simulink model "TransmissionDownshift"  (R2022a)
settings: Solver=ode5  StartTime=0.0  StopTime=100  RelTol=1e-3  AbsTol=1e-6
model workspace (MAT data in the model file):
  Iei = 0.0219914882836
  converter_data = [0  137.465208994  2.232; 0.1  137.065019157  2.075; 0.2  135.864449646  1.975; 0.3  135.664354728  1.846; 0.4  137.565256453  1.72; 0.5  140.366585312  1.564; 0.6  145.268910814  1.409; 0.7  152.872517717  1.254; 0.8  162.9773111  1.096; 0.81  164.27792807  1.08; 0.82  166.178829795  1.061; 0.83  167.979684062  1.043; 0.84  170.080680706  1.028; 0.85  172.781962105  1.012; 0.86  175.383196045  1.002; 0.87  179.585189333  1.002; 0.88  183.587087703  1.001; 0.89  189.890077635  0.998; 0.9  197.693779455  0.999; 0.92  215.902417037  1.001; 0.94  244.515990379  1.002]
  downtab = [0  5  20  35; 0  5  20  35; 0  5  25  40; 0  5  30  50; 0  30  50  80; 0  30  50  80]
  downth = [0; 5; 40; 50; 90; 100]
  emap = [-40  -44  -49  -53  -57  -61  -65  -70  -74  -78  -82; 215  117  85  66  44  29  10  -2  -13  -22  -32; 245  208  178  148  122  104  85  66  48  33  18; 264  260  241  219  193  167  152  133  119  96  85; 264  279  282  275  260  238  223  208  189  171  152; 267  290  293  297  290  275  260  256  234  212  193; 267  297  305  305  305  301  293  282  267  249  226; 267  301  308  312  319  323  319  316  297  279  253; 267  301  312  319  327  327  327  327  312  293  267; 267  301  312  319  327  334  334  334  319  305  275]
  nevec = [800 1200 1600 2000 2400 2800 3200 3600 4000 4400 4800]
  p0 = 0.07934
  p1 = 0.07934
  thvec = [0; 20; 30; 40; 50; 60; 70; 80; 90; 100]
  uptab = [10  30  50  1000000; 10  30  50  1000000; 15  30  50  1000000; 23  41  60  1000000; 40  70  100  1000000; 40  70  100  1000000]
  upth = [0; 25; 35; 50; 90; 100]
  vehicledata = [3.23; 40; 0.3; 1; 50; 0]
undefined symbols (not defined in the file or in its folder): gearType, Hecate_Param1, Hecate_Param2, Hecate_Param3, Hecate_Param4
Description:
  | TransmissionDownshiftTestSequence model
  | The model is used to show how to test a transmission shift logic controller using test sequences and assessments.
settings Model: ExtModeTrigMode=oneshot  ExtModeArmWhenConnect=off  Creator=The MathWorks, Inc.  LastModifiedBy=admin
settings SolverCC: AutoScaleAbsTol=off  AlgebraicLoopSolver=TrustRegion  MaxZcPerStep=1
settings DataIOCC: InitialState=X0  LoadInitialState=on  SaveFormat=Structure  ReturnWorkspaceOutputs=off  SignalLoggingName=sigsOut
settings OptimizationCC: BlockReduction=off  BooleanDataType=off  DefaultParameterBehavior=Inlined  ExpressionDepthLimit=2147483647  InitFltsAndDblsToZero=on  EfficientMapNaN2IntZero=off  LifeSpan=1  EfficientTunableParamExpr=on
settings DebuggingCC: SaveWithParameterizedLinksMsg=none  UnderspecifiedInitializationDetection=Classic  MergeDetectMultiDrivingBlocksExec=none  CheckExecutionContextPreStartOutputMsg=on  SignalResolutionControl=TryResolveAllWithWarning  MultiTaskDSMMsg=warning  MultiTaskCondExecSysMsg=none  IntegerOverflowMsg=none  FcnCallInpInsideContextMsg=warning  UnconnectedInputMsg=warning  UnconnectedOutputMsg=warning  UnconnectedLineMsg=warning  AllowSymbolicDim=off  StateNameClashWarn=warning  SFUnexpectedBacktrackingDiag=warning  SFNoUnconditionalDefaultTransitionDiag=warning  SFExecutionAtInitializationDiag=none  SFMachineParentedDataDiag=warning  IntegerSaturationMsg=none  ArithmeticOperatorsInVariantConditions=warning
settings HardwareCC: ProdBitPerPointer=32  ProdBitPerSizeT=32  ProdBitPerPtrDiffT=32  ProdLargestAtomicFloat=None  ProdIntDivRoundTo=Undefined  ProdEndianess=Unspecified  ProdWordSize=32  ProdHWDeviceType=32-bit Generic  TargetBitPerLong=64  TargetBitPerPointer=64  TargetBitPerSizeT=64  TargetBitPerPtrDiffT=64  TargetLongLongMode=on  TargetIntDivRoundTo=Zero  TargetEndianess=LittleEndian  TargetWordSize=64  TargetHWDeviceType=MATLAB Host  ProdEqTarget=off
settings ModelReferenceCC: PropagateSignalLabelsOutOfModel=off
settings SFSimCC: SFSimEcho=off  SimUseLocalCustomCode=off  SimParseCustomCode=off  MATLABDynamicMemAlloc=off  CustomCodeUndefinedFunction=UseInterfaceOnly
settings RTWCC: SystemTargetFile=ert.tlc  TemplateMakefile=ert_default_tmf  RTWUseLocalCustomCode=off  DLArmComputeVersion=19.05
settings CodeAppCC: IgnoreCustomStorageClasses=off  CustomSymbolStrModelFcn=$N  StateflowObjectComments=on
settings ERTTargetCC: MultiwordLength=2048  GenerateSampleERTMain=on  InlinedParameterPlacement=NonHierarchical  ERTCustomFileTemplate=example_file_process.tlc  ConvertIfToSwitch=off  SuppressUnreachableDefaultCases=off
settings ConfigComp: CovMetricSettings=dcmtr  CovSaveCumulativeToWorkspaceVar=on  CovSaveSingleToWorkspaceVar=on  CovExternalEMLEnable=off  CovSFcnEnable=off

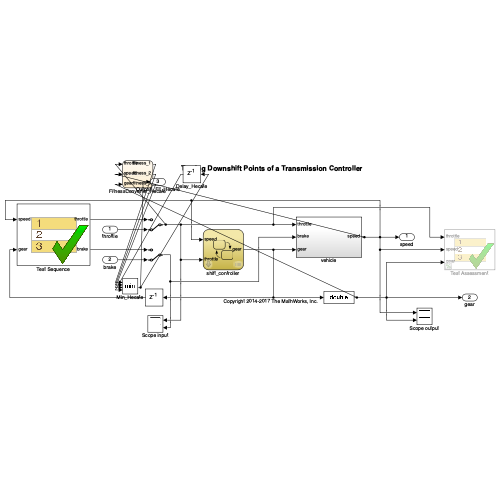
[thumbnail: Simulink's stored preview of the top-level diagram]
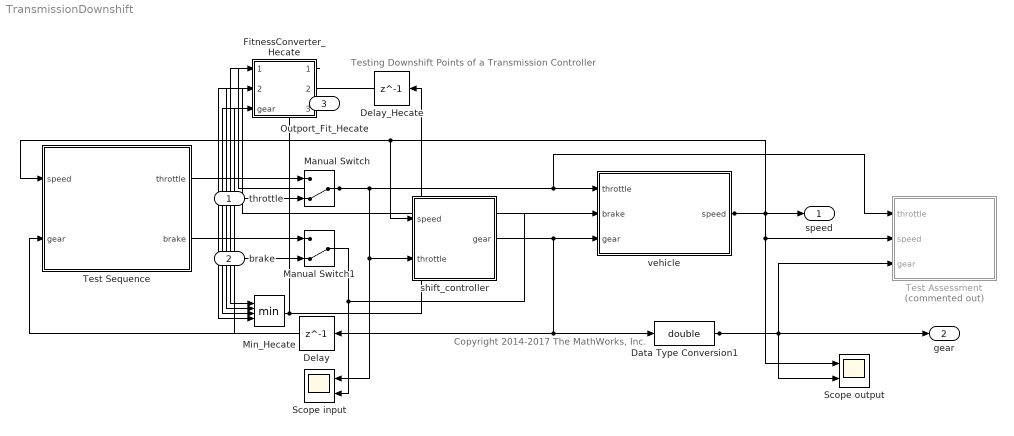
== system TransmissionDownshift ==
  note: Copyright 2014-2017 The MathWorks, Inc.
  note: Testing Downshift Points of a Transmission Controller
  throttle : Inport
  brake : Inport  Port=2
  Data Type Conversion1 : DataTypeConversion  OutDataTypeStr=double  SaturateOnIntegerOverflow=off  RndMeth=Floor
  Delay : Delay  DelayLength=1  InitialCondition=gearType.first
  Delay_Hecate : Delay  DelayLength=1  InitialCondition=Inf
  FitnessConverter_Hecate : Stateflow chart  TreatAsAtomicUnit=on
  Manual Switch : ManualSwitch  CurrentSetting=0
  Manual Switch1 : ManualSwitch  CurrentSetting=0
  Min_Hecate : MinMax  Inputs=4
  Scope input : Scope  NumInputPorts=2
  Scope output : Scope  NumInputPorts=2
  Test Assessment : Test Sequence  Tag=__SLT_ASMT__  Commented=on  TreatAsAtomicUnit=on
  Test Sequence : Test Sequence  TreatAsAtomicUnit=on
  shift_controller : Stateflow chart  TreatAsAtomicUnit=on  mask{TWAIT=2}
      mask prompts: TWAIT "Delay before gear change (tick)"
  vehicle : Subsystem
  speed : Outport  VectorParamsAs1DForOutWhenUnconnected=off
  gear : Outport  Port=2  VectorParamsAs1DForOutWhenUnconnected=off
  Outport_Fit_Hecate : Outport  Port=3
  wires:
  vehicle/1(speed) -> speed/1, Test Assessment/2(speed), Scope output/1, Test Sequence/1(speed), shift_controller/1(speed), FitnessConverter_Hecate/2(speed)
  Test Sequence/2(brake) -> Manual Switch1/1
  Test Sequence/1(throttle) -> Manual Switch/1
  throttle/1 -> Manual Switch/2
  brake/1 -> Manual Switch1/2
  Manual Switch/1 -> vehicle/1(throttle), Test Assessment/1(throttle), Scope input/1, shift_controller/2(throttle), FitnessConverter_Hecate/1(throttle)
  Manual Switch1/1 -> vehicle/2(brake), Scope input/2
  Delay/1 -> Test Sequence/2(gear)
  shift_controller/1(" gear") -> Delay/1, Data Type Conversion1/1, vehicle/3(gear)
  Data Type Conversion1/1 -> Test Assessment/3(gear), gear/1, Scope output/2, FitnessConverter_Hecate/3(gear)
  FitnessConverter_Hecate/1(fitness_1) -> Min_Hecate/1
  FitnessConverter_Hecate/2(fitness_2) -> Min_Hecate/2
  FitnessConverter_Hecate/3(fitness_3) -> Min_Hecate/3
  Min_Hecate/1 -> Delay_Hecate/1, Outport_Fit_Hecate/1
  Delay_Hecate/1 -> Min_Hecate/4

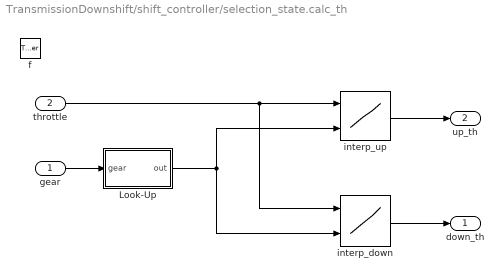
== system TransmissionDownshift/shift_controller/selection_state.calc_th ==
  gear : Inport  OutDataTypeStr=Enum: gearType  PortDimensions=1
  throttle : Inport  Port=2  OutDataTypeStr=double  PortDimensions=1
  f : TriggerPort  TriggerType=function-call  VariantControl=Variant
      settings: CopyFcn=Stateflow.SLINSF.SimulinkMan.removeBlockPreDeleteFcn  PreDeleteFcn=Stateflow.SLINSF.SimulinkMan.unsafePredeleteFcn
  Look-Up : MATLAB Function  TreatAsAtomicUnit=on
  interp_down : Lookup_n-D  BreakpointsForDimension1=downth  BreakpointsForDimension2=[1:4]  Table=downtab
      settings: InputPortMap=u0,u1
  interp_up : Lookup_n-D  BreakpointsForDimension1=upth  BreakpointsForDimension2=[1:4]  Table=uptab
      settings: InputPortMap=u0,u1
  down_th : Outport  VectorParamsAs1DForOutWhenUnconnected=off
  up_th : Outport  Port=2  VectorParamsAs1DForOutWhenUnconnected=off
  wires:
  interp_up/1 -> up_th/1
  interp_down/1 -> down_th/1
  throttle/1 -> interp_down/1, interp_up/1
  gear/1 -> Look-Up/1(gear)
  Look-Up/1(out) -> interp_down/2, interp_up/2

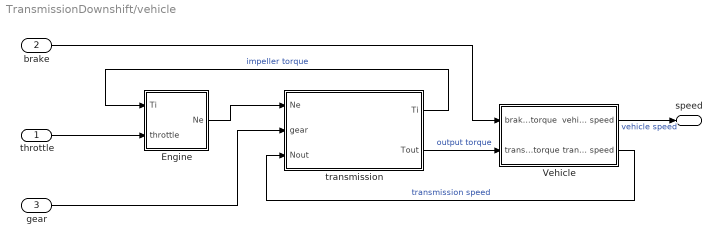
== system TransmissionDownshift/vehicle ==
  throttle : Inport
  brake : Inport  Port=2
  gear : Inport  Port=3
  Engine : Subsystem
  Vehicle : Subsystem  mask(vehicle model){Rfd=vehicledata(1), rload0=vehicledata(2), rload2=vehicledata(3), Rw=vehicledata(4), Iv=vehicledata(5), N20=vehicledata(6)/vehicledata(4)*vehicledata(1)}
      mask prompts: Rfd "final drive ratio"; rload0 "drag friction at wheels"; rload2 "aerodynamic drag"; Rw "wheel radius"; Iv "vehicle inertia"; N20 "initial transmission output speed"
      mask help: vehicle dynamics: torque input from trans., outputs are input speed (transmission output) and vehicle speed
      mask Display: image('NSX_3Colors.jpg')
  transmission : Subsystem
      mask Display:
      | image('transmission_diagram.svg')
      | port_label('input', 1, 'Ne')
      | port_label('input', 2, 'gear')
      | port_label('input', 3, 'Nout')
      | port_label('output', 1, 'Ti')
      | port_label('output', 2, 'Tout')
  speed : Outport  VectorParamsAs1DForOutWhenUnconnected=off
  wires:
  throttle/1 -> Engine/2(throttle)
  transmission/1(Ti) -> Engine/1(Ti)  "impeller torque"
  Engine/1(Ne) -> transmission/1(Ne)
  transmission/2(Tout) -> Vehicle/2(transmission output torque)  "output torque"
  Vehicle/2(transmission output speed) -> transmission/3(Nout)  "transmission speed"
  Vehicle/1(vehicle speed) -> speed/1  "vehicle speed"
  brake/1 -> Vehicle/1(brake torque)
  gear/1 -> transmission/2(gear)

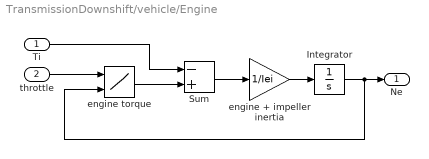
== system TransmissionDownshift/vehicle/Engine ==
  Ti : Inport
  throttle : Inport  Port=2
  Integrator : Integrator  InitialCondition=1000  LimitOutput=on  UpperSaturationLimit=6000  LowerSaturationLimit=600  ZeroCross=off
  Sum : Sum  Inputs=-+  InputSameDT=on  SaturateOnIntegerOverflow=on  OutDataTypeStr=Inherit: Same as first input
  engine torque : Lookup_n-D  BreakpointsForDimension1=thvec  BreakpointsForDimension2=nevec  Table=emap  InternalRulePriority=Speed
      settings: InputPortMap=u0,u1
  engine + impeller inertia : Gain  Gain=1/Iei  SaturateOnIntegerOverflow=on  OutDataTypeStr=Inherit: Same as input  ParamDataTypeStr=Inherit: Same as input
  Ne : Outport  VectorParamsAs1DForOutWhenUnconnected=off
  wires:
  Ti/1 -> Sum/1
  throttle/1 -> engine torque/1
  Integrator/1 -> engine torque/2, Ne/1
  Sum/1 -> engine + impeller inertia/1
  engine + impeller inertia/1 -> Integrator/1
  engine torque/1 -> Sum/2

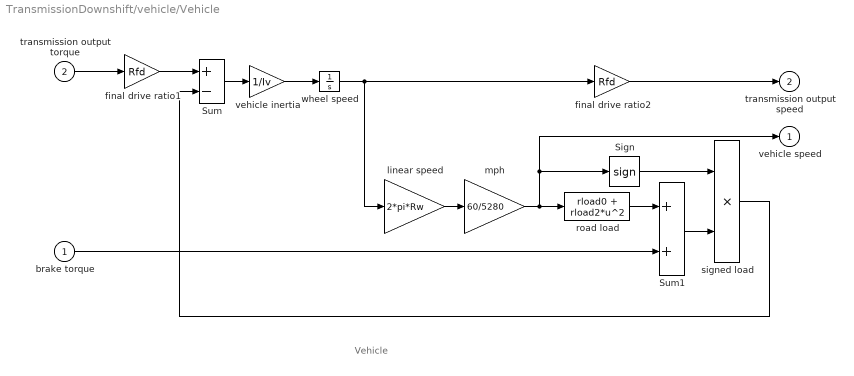
== system TransmissionDownshift/vehicle/Vehicle ==
  note: Vehicle
  brake torque : Inport
  transmission output torque : Inport  Port=2
  Sign : Signum
  Sum : Sum  Inputs=+-  InputSameDT=on  SaturateOnIntegerOverflow=on  OutDataTypeStr=Inherit: Same as first input
  Sum1 : Sum  InputSameDT=on  SaturateOnIntegerOverflow=on  OutDataTypeStr=Inherit: Same as first input
  final drive ratio1 : Gain  Gain=Rfd  SaturateOnIntegerOverflow=on  OutDataTypeStr=Inherit: Same as input  ParamDataTypeStr=Inherit: Same as input
  final drive ratio2 : Gain  Gain=Rfd  SaturateOnIntegerOverflow=on  OutDataTypeStr=Inherit: Same as input  ParamDataTypeStr=Inherit: Same as input
  linear speed : Gain  Gain=2*pi*Rw  SaturateOnIntegerOverflow=on  OutDataTypeStr=Inherit: Same as input  ParamDataTypeStr=Inherit: Same as input
  mph : Gain  Gain=60/5280  SaturateOnIntegerOverflow=on  OutDataTypeStr=Inherit: Same as input  ParamDataTypeStr=Inherit: Same as input
  road load : Fcn  Expr=rload0 + rload2*u^2
  signed load : Product  InputSameDT=on  SaturateOnIntegerOverflow=on  OutDataTypeStr=Inherit: Same as first input
  vehicle inertia : Gain  Gain=1/Iv  SaturateOnIntegerOverflow=on  OutDataTypeStr=Inherit: Same as input  ParamDataTypeStr=Inherit: Same as input
  wheel speed : Integrator  InitialCondition=N20/Rfd  ZeroCross=off
  vehicle speed : Outport  VectorParamsAs1DForOutWhenUnconnected=off
  transmission output speed : Outport  Port=2  VectorParamsAs1DForOutWhenUnconnected=off
  wires:
  final drive ratio2/1 -> transmission output speed/1
  brake torque/1 -> Sum1/2
  Sum1/1 -> signed load/2
  road load/1 -> Sum1/1
  Sign/1 -> signed load/1
  signed load/1 -> Sum/2
  transmission output torque/1 -> final drive ratio1/1
  vehicle inertia/1 -> wheel speed/1
  Sum/1 -> vehicle inertia/1
  mph/1 -> vehicle speed/1, Sign/1, road load/1
  linear speed/1 -> mph/1
  wheel speed/1 -> linear speed/1, final drive ratio2/1
  final drive ratio1/1 -> Sum/1

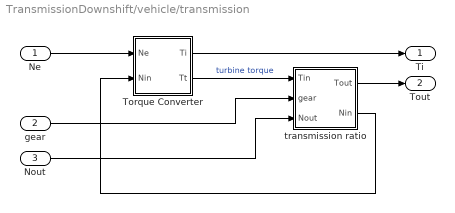
== system TransmissionDownshift/vehicle/transmission ==
  Ne : Inport
  gear : Inport  Port=2
  Nout : Inport  Port=3
  Torque Converter : Subsystem  mask(torque converter){speedratio=converter_data(:,1), Kfactor=converter_data(:,2), Torkratio=converter_data(:,3)}
      mask prompts: speedratio "speed ratio"; Kfactor "K factor"; Torkratio "torque ratio"
      mask help: torque converter
      mask Help: Torque converter input and output torques are computed as a function of the input and output speeds
      mask Display: plot([cos([90:10:450]*pi/180),.63*cos([90:10:450]*pi/180),.63*cos([90:10:240]*pi/180),cos([240:10:300]*pi/180),.63*cos([300]*pi/180)],[sin([90:10:450]*pi/180),.63*sin([90:10:450]*pi/180)+.1,.63*sin([90:10:240]*pi/180)+.1,sin([240:10:300]*pi/180),.63*sin([300]*pi/180)+.1])
  transmission ratio : Subsystem
  Ti : Outport  VectorParamsAs1DForOutWhenUnconnected=off
  Tout : Outport  Port=2  VectorParamsAs1DForOutWhenUnconnected=off
  wires:
  transmission ratio/1(Tout) -> Tout/1
  Torque Converter/1(Ti) -> Ti/1
  Nout/1 -> transmission ratio/3(Nout)
  gear/1 -> transmission ratio/2(gear)
  Ne/1 -> Torque Converter/1(Ne)
  transmission ratio/2(Nin) -> Torque Converter/2(Nin)
  Torque Converter/2(Tt) -> transmission ratio/1(Tin)  "turbine torque"

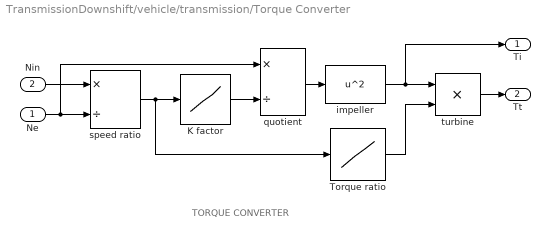
== system TransmissionDownshift/vehicle/transmission/Torque Converter ==
  note: TORQUE CONVERTER
  Ne : Inport
  Nin : Inport  Port=2
  K factor : Lookup_n-D  NumberOfTableDimensions=1  BreakpointsForDimension1=speedratio  Table=Kfactor  InternalRulePriority=Speed  SaturateOnIntegerOverflow=on
  Torque ratio : Lookup_n-D  NumberOfTableDimensions=1  BreakpointsForDimension1=speedratio  Table=Torkratio  InternalRulePriority=Speed  SaturateOnIntegerOverflow=on
  impeller : Fcn  Expr=u^2
  quotient : Product  Inputs=*/  InputSameDT=on  SaturateOnIntegerOverflow=on  OutDataTypeStr=Inherit: Same as first input
  speed ratio : Product  Inputs=*/  InputSameDT=on  SaturateOnIntegerOverflow=on  OutDataTypeStr=Inherit: Same as first input
  turbine : Product  InputSameDT=on  SaturateOnIntegerOverflow=on  OutDataTypeStr=Inherit: Same as first input
  Ti : Outport  VectorParamsAs1DForOutWhenUnconnected=off
  Tt : Outport  Port=2  VectorParamsAs1DForOutWhenUnconnected=off
  wires:
  Torque ratio/1 -> turbine/2
  quotient/1 -> impeller/1
  K factor/1 -> quotient/2
  speed ratio/1 -> Torque ratio/1, K factor/1
  impeller/1 -> turbine/1, Ti/1
  turbine/1 -> Tt/1
  Ne/1 -> speed ratio/2, quotient/1
  Nin/1 -> speed ratio/1

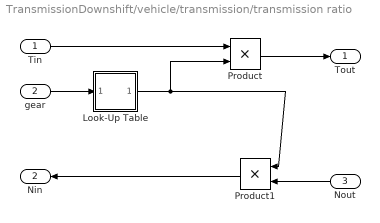
== system TransmissionDownshift/vehicle/transmission/transmission ratio ==
  Tin : Inport
  gear : Inport  Port=2
  Nout : Inport  Port=3
  Look-Up Table : MATLAB Function  TreatAsAtomicUnit=on
  Product : Product  InputSameDT=on  SaturateOnIntegerOverflow=on  OutDataTypeStr=Inherit: Same as first input
  Product1 : Product  InputSameDT=on  SaturateOnIntegerOverflow=on  OutDataTypeStr=Inherit: Same as first input
  Tout : Outport  VectorParamsAs1DForOutWhenUnconnected=off
  Nin : Outport  Port=2  VectorParamsAs1DForOutWhenUnconnected=off
  wires:
  Look-Up Table/1(out) -> Product1/1, Product/2
  Nout/1 -> Product1/2
  Product1/1 -> Nin/1
  Product/1 -> Tout/1
  Tin/1 -> Product/1
  gear/1 -> Look-Up Table/1(gear)

== matlab function TransmissionDownshift/vehicle/transmission/transmission ratio/Look-Up Table ==
  data: gear input; out output
function out = fcn(gear)
    %#codegen
    table = [2.393 1.450 1.000 0.677];
    switch(gear)
        case gearType.fourth
            out=table(4);        
        case gearType.third
            out=table(3);            
        case gearType.second
            out=table(2);
        otherwise % gearType.first
            out=table(1);
    end
    
end

== stateflow chart TransmissionDownshift/FitnessConverter_Hecate ==
  state AssertConditions
    fitness_1 = Inf;
    fitness_2 = Inf;
    fitness_3 = Inf;
    state OverSpeed3
      fitness_1 = 90-(speed);
      fitness_2 = Inf;
      fitness_3 = Inf;
    state OverSpeed2
      fitness_1 = Inf;
      fitness_2 = 50-(speed);
      fitness_3 = Inf;
    state OverSpeed1
      fitness_1 = Inf;
      fitness_2 = Inf;
      fitness_3 = 30-(speed);
    state Else
      fitness_1 = Inf;
      fitness_2 = Inf;
      fitness_3 = Inf;
    (default) -> (junction 4)
    Else -> (junction 4) : [(gear==3)|(gear==2)|(gear==1)]
    OverSpeed1 -> (junction 4) : [(gear==3)|(gear==2)|~(gear==1)]
    OverSpeed2 -> (junction 4) : [(gear==3)|~(gear==2)]
    (junction 4) -> OverSpeed3 [order 1] : [gear==3]
    (junction 4) -> OverSpeed2 [order 2] : [gear==2]
    (junction 4) -> OverSpeed1 [order 3] : [gear==1]
    (junction 4) -> Else [order 4] : []
    OverSpeed3 -> (junction 4) : [~(gear==3)]
  (default) -> AssertConditions
  data: throttle input; speed input; gear input; fitness_1 output; fitness_2 output; fitness_3 output

== stateflow chart TransmissionDownshift/Test Sequence ==
  settings: stateMachineType=SIMPLIFIED_MACHINE
  state AT2_1
    state Step1
      throttle = 50+Hecate_Param1;
      brake = 50+Hecate_Param2;
    state Step2
      throttle = 50+Hecate_Param3;
      brake = 50+Hecate_Param4;
    (default) -> Step1
    Step1 -> Step2 : [
        | et(sec)>20
        | ]
  state AT2_2
    state Accelerate
      throttle = 100;
      brake = 0;
    state Stop
      throttle = 0;
      brake = 325;
    (default) -> Accelerate
    Accelerate -> Stop : [
        | duration(gear == 4) >= Limit
        | ]
  (default) -> AT2_1 [order 1] : [Active_Scenario_Index == 1]
  (default) -> AT2_2 [order 2] : {assert(Active_Scenario_Index == 2,'The value of Scenario Parameter ''Active_Scenario_Index'' is not valid. Use the index of the scenario to specify it.')}
  data: speed input; gear input; throttle output double; brake output double; Active_Scenario_Index parameter =1; Limit constant double =2; Hecate_Param3 parameter; Hecate_Param2 parameter; Hecate_Param1 parameter; Hecate_Param4 parameter

== stateflow chart TransmissionDownshift/Test Assessment ==
  settings: stateMachineType=SIMPLIFIED_MACHINE
  state AT2_1
    state AssertConditions
      % These conditions ensure simulation validity.
      %assert(speed >= 0, 'speed must be >= 0');
      %assert(gear > 0,'gear must be > 0');
      state OverSpeed3
        % Verify speed within specified range for 3rd gear
        verify(speed <= 90,'Engine overspeed in gear 3')
      state OverSpeed2
        % Verify speed within specified range for 2nd gear
        verify(speed <=50,'Engine overspeed in gear 2')
      state OverSpeed1
        % Verify speed within specified range for 1st gear
        verify(speed <= 30,'Engine overspeed in gear 1')
      state Else
        % Else step required for any conditions not corresponding to
        % the above three when conditions
      (default) -> (junction 83)
      AssertConditions -> (junction 83)
      (junction 83) -> (junction 84) [order 1] : [gear==3
          | ]
      (junction 84) -> OverSpeed3 [order 1] : [~in(AT2_1.AssertConditions.OverSpeed3)]
      (junction 83) -> (junction 93) [order 2]
      (junction 84) -> (junction 87) [order 2]
      (junction 93) -> (junction 94) [order 1] : [gear==2
          | ]
      (junction 94) -> OverSpeed2 [order 1] : [~in(AT2_1.AssertConditions.OverSpeed2)]
      (junction 93) -> (junction 101) [order 2]
      (junction 94) -> (junction 97) [order 2]
      (junction 101) -> (junction 102) [order 1] : [gear==1
          | ]
      (junction 102) -> OverSpeed1 [order 1] : [~in(AT2_1.AssertConditions.OverSpeed1)]
      (junction 101) -> (junction 109) [order 2]
      (junction 102) -> (junction 105) [order 2]
      (junction 109) -> (junction 110)
      (junction 110) -> AT2_1.AssertConditions.Else [order 1] : [~in(AT2_1.AssertConditions.Else)]
      (junction 110) -> (junction 113) [order 2]
    (default) -> AssertConditions
  state AT2_2
    state Assessments
      state Check1st
        verify(speed < 45)
      state Check2nd
        verify(speed < 75)
      state Check3rd
        verify(speed < 105)
      state Else
      Assessments -> (junction 129)
      (default) -> (junction 129)
      (junction 129) -> (junction 130) [order 1] : [gear == 1
          | ]
      (junction 130) -> Check1st [order 1] : [~in(AT2_2.Assessments.Check1st)]
      (junction 129) -> (junction 143) [order 2]
      (junction 130) -> (junction 133) [order 2]
      (junction 143) -> (junction 144) [order 1] : [gear == 2
          | ]
      (junction 144) -> Check2nd [order 1] : [~in(AT2_2.Assessments.Check2nd)]
      (junction 143) -> (junction 151) [order 2]
      (junction 144) -> (junction 147) [order 2]
      (junction 151) -> (junction 152) [order 1] : [gear == 3
          | ]
      (junction 152) -> Check3rd [order 1] : [~in(AT2_2.Assessments.Check3rd)]
      (junction 152) -> (junction 155) [order 2]
      (junction 159) -> (junction 160)
      (junction 160) -> AT2_2.Assessments.Else [order 1] : [~in(AT2_2.Assessments.Else)]
      (junction 160) -> (junction 163) [order 2]
      (junction 151) -> (junction 159) [order 2]
    (default) -> Assessments
  (default) -> AT2_1 [order 1] : [Active_Scenario_Index == 1]
  (default) -> AT2_2 [order 2] : {assert(Active_Scenario_Index == 2,'The value of Scenario Parameter ''Active_Scenario_Index'' is not valid. Use the index of the scenario to specify it.')}
  data: throttle input; speed input; gear input; Active_Scenario_Index parameter =1

== stateflow chart TransmissionDownshift/shift_controller ==
  settings: updateMethod=DISCRETE  sampleTime=0.04
  state gear_state [parallel]
    settings: executionOrder=1
    state fourth
    state third
    state second
    state first
    (default) -> first
    second -> third [order 1] : UP
    third -> fourth [order 1] : UP
    first -> second : UP
    fourth -> third : DOWN
    third -> second [order 2] : DOWN
    second -> first [order 2] : DOWN
  state selection_state [parallel]
    during: [down_th,up_th] = calc_th(gear,throttle);
    settings: executionOrder=2
    state steady_state
    state upshifting
    state downshifting
    state [down_th,up_th] = calc_th(gear,throttle) [function]
    (default) -> steady_state
    steady_state -> upshifting [order 1] : [speed > up_th]
    steady_state -> downshifting [order 2] : [speed < down_th]
    downshifting -> steady_state [order 1] : after(TWAIT,tick)
        | [speed <= down_th]
        | {gear_state.DOWN}
    downshifting -> steady_state [order 2] : [speed > down_th]
    upshifting -> steady_state [order 1] : after(TWAIT,tick)
        | [speed >= up_th]
        | {gear_state.UP}
    upshifting -> steady_state [order 2] : [speed < up_th]
  data: gear function_input Enum: gearType size=1; throttle function_input double size=1; down_th function_output; up_th function_output; speed input double; TWAIT parameter uint8; up_th local double; down_th local double; throttle input; gear output Enum: gearType
  events: DOWN local EITHER_EDGE_EVENT; UP local EITHER_EDGE_EVENT

== matlab function TransmissionDownshift/shift_controller/selection_state.calc_th/Look-Up ==
  data: gear input; out output
function out = fcn(gear)
    %#codegen
    table = [1 2 3 4];
    switch(gear)
        case gearType.fourth;
            out=table(4);        
        case gearType.third;
            out=table(3);
        case gearType.second;
            out=table(2);            
        otherwise; % gearType.first
            out=table(1);
    end
    
end
